simulink model "simulinkex5l3"  (R2022b)
settings: Solver=VariableStepAuto  StartTime=0.0  StopTime=10.0  RelTol=1e-3
libraries: simulink x1
settings Model: Creator=gokuz  LastModifiedBy=gokuz

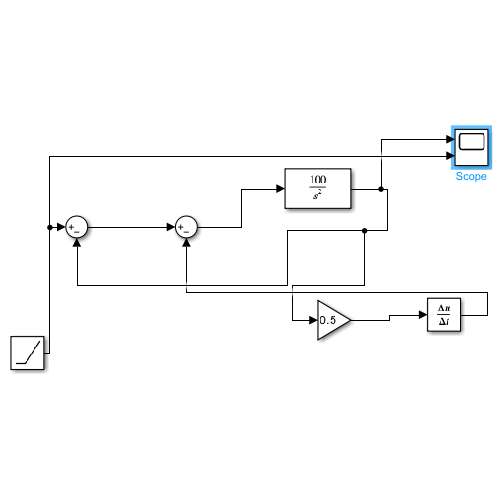
[thumbnail: Simulink's stored preview of the top-level diagram]
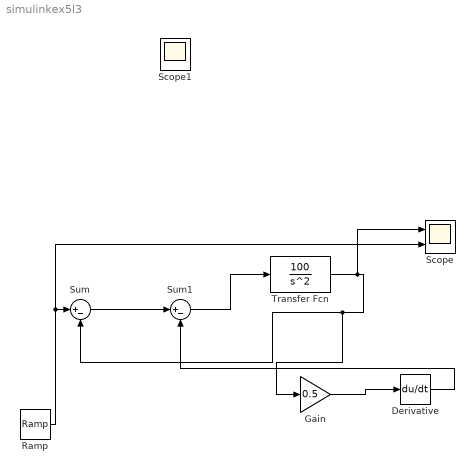
== system simulinkex5l3 ==
  Derivative : Derivative  CoefficientInTFapproximation=0
  Gain : Gain  Gain=0.5
  Ramp : simulink/Sources/Ramp  slope=1  start=0  InitialOutput=0
  Scope : Scope  NumInputPorts=2
  Sum : Sum  Inputs=|+-
  Sum1 : Sum  Inputs=|+-
  Transfer Fcn : TransferFcn  Numerator=[0 100]  Denominator=[1 0 0]
  Scope1 : Scope
  wires:
  Ramp/1 -> Scope/2, Sum/1
  Sum/1 -> Sum1/1
  Transfer Fcn/1 -> Scope/1, Sum/2, Gain/1
  Sum1/1 -> Transfer Fcn/1
  Gain/1 -> Derivative/1
  Derivative/1 -> Sum1/2
